simulink model "Masse_MultirotorSimHinf"  (R2018b)
(part 5 of 11)

	% float
	betaTmp = (r' * (S_I * r));
	beta1 = betaTmp(1, 1);

	if (beta1 > self.BETA_TABLE(n_y_baro) )
		if (~bitand(self.sensorFault, self.SENSOR_BARO))
			% mavlink_log_critical(&mavlink_log_pub, '[lpe] baro fault, r %5.2f m, beta1 %5.2f', ...
			% 		     double(r(0)), double(beta1));
			self.sensorFault = bitor( self.sensorFault, self.SENSOR_BARO );
		end

    elseif bitand(self.sensorFault, self.SENSOR_BARO)
		self.sensorFault = bitand( self.sensorFault, bitcmp( self.SENSOR_BARO , 'uint8' ));
		% mavlink_and_console_log_info(mavlink_log_pub, '[lpe] baro OK');
	end

	% kalman filter correction always
	%Matrix<float, n_x, n_y_baro>
	K = self.P * C' * S_I;
	%Vector<float, n_x>
	dx = K * r;
	self.x = self.x + dx;
	self.P = self.P - K * C * self.P;
end

% void BlockLocalPositionEstimator::
function self = baroCheckTimeout( self )
%BAROCHECKTIMEOUT Check barometer timeout
	BARO_TIMEOUT = 100000;
	if ( (self.timeStamp - self.time_last_baro) > BARO_TIMEOUT)
		if (~bitand(self.sensorTimeout, self.SENSOR_BARO))
			self.sensorTimeout = bitor( self.sensorTimeout, self.SENSOR_BARO );
			self.baroStats.count = 0;
			self.baroStats.total = 0;
			% mavlink_and_console_log_info(mavlink_log_pub, '[lpe] baro timeout ');
		end
	end
end

%% LAND
% void BlockLocalPositionEstimator::
function self = landInit( self )
	% measure
    REQ_LAND_INIT_COUNT = 1;
	% Vector<float, n_y_land> y;

    [ self, landOk, ~ ] = landMeasure( self );
	if ( landOk ~= 1)
		self.landCount = 0;
	end

	% if finished
	if (self.landCount > REQ_LAND_INIT_COUNT)
		% mavlink_and_console_log_info(mavlink_log_pub, '[lpe] land init');
		self.sensorTimeout = bitand( self.sensorTimeout, bitcmp(self.SENSOR_LAND, 'uint8') );
		self.sensorFault   = bitand( self.sensorFault,   bitcmp(self.SENSOR_LAND, 'uint8' ) );
	end
end

% int BlockLocalPositionEstimator::
function [ self, output, y ] = landMeasure( self )
    Y_land_vx = 1; Y_land_vy = 2; Y_land_agl = 3; n_y_land = 3;
    
	self.time_last_land = self.timeStamp;
	y = zeros( n_y_land, 1 ); %.setZero();
	self.landCount = self.landCount + 1;
	output = 1;
end

%void BlockLocalPositionEstimator::
function self = landCorrect( self )
	% measure land
    X_x = 1; X_y = 2; X_z = 3; X_vx = 4; X_vy = 5; X_vz = 6;
	X_bx = 7; X_by = 8; X_bz = 9; X_tz = 10; n_x = 10;
    Y_land_vx = 1; Y_land_vy = 2; Y_land_agl = 3; n_y_land = 3;
	y = zeros( n_y_land, 1);

    [ self, landOk, y ] = landMeasure( self );
	if ( landOk ~= 1)
		return;
	end

	% measurement matrix
	% Matrix<float, n_y_land, n_x> C;
	C = zeros( n_y_land, n_x );
	% y = -(z - tz)
	C(Y_land_vx, X_vx) = 1;
	C(Y_land_vy, X_vy) = 1;
	C(Y_land_agl, X_z) = -1; % measured altitude, negative down dir.
	C(Y_land_agl, X_tz) = 1; % measured altitude, negative down dir.

	% use parameter covariance
	% SquareMatrix<float, n_y_land> R;
	R = zeros( n_y_land, n_y_land );
	R(Y_land_vx, Y_land_vx) = self.land_vxy_stddev * self.land_vxy_stddev;
	R(Y_land_vy, Y_land_vy) = self.land_vxy_stddev * self.land_vxy_stddev;
	R(Y_land_agl, Y_land_agl) = self.land_z_stddev * self.land_z_stddev;

	% residual
	%Matrix<float, n_y_land, n_y_land> S_I = inv<float, n_y_land>((C * self.P * C.transpose()) + R);
	%Vector<float, n_y_land> r = y - C * self.x;
    S_I = inv((C * self.P * C') + R);
	r = y - (C * self.x);
	self.pub_innov.hagl_innov     = r(Y_land_agl);
	self.pub_innov.hagl_innov_var = R(Y_land_agl, Y_land_agl);

	% fault detection
    betaTmp = (r' * (S_I * r));
	beta1 = betaTmp(1, 1);

	% artifically increase beta threshhold to prevent fault during landing
	beta_thresh = 1e2;

	if ( (beta1 / self.BETA_TABLE(n_y_land)) > beta_thresh)
		if ( ~bitand(self.sensorFault, self.SENSOR_LAND) )
			self.sensorFault = bitor( self.sensorFault, self.SENSOR_LAND);
			% mavlink_and_console_log_info(&mavlink_log_pub, '[lpe] land fault,  beta %5.2f', double(beta));
		end

		% abort correction
		return;

    elseif bitand(self.sensorFault, self.SENSOR_LAND)
		self.sensorFault = bitand( self.sensorFault, bitcmp( self.SENSOR_LAND, 'uint8' ));
		% mavlink_and_console_log_info(mavlink_log_pub, '[lpe] land OK');
	end

	% kalman filter correction always for land detector
	% Matrix<float, n_x, n_y_land>
    K = self.P * C' * S_I;
	% Vector<float, n_x>
    dx = K * r;
	self.x = self.x + dx;
	self.P = self.P - K * C * self.P;
end

%void BlockLocalPositionEstimator::
function self = landCheckTimeout( self )
    LAND_TIMEOUT =   1000000; % 1.0 s
	if ( (self.timeStamp - self.time_last_land) > LAND_TIMEOUT)
		if (~bitand(self.sensorTimeout, self.SENSOR_LAND))
			self.sensorTimeout = bitor( self.sensorTimeout, self.SENSOR_LAND);
			self.landCount = 0;
			% mavlink_and_console_log_info(&mavlink_log_pub, '[lpe] land timeout ');
		end
	end
end
